simulink model "subsystem1"  (R2023a)
settings: Solver=VariableStepAuto  StartTime=0.0  StopTime=10  RelTol=1e-3  AbsTol=1e-3
values from neighbouring files (symbols this model uses):
  b = 1    [KATSAYI.m]    (also in hiz.m = 0.1; kat.m = 0.1; matlab.mat; untitled.m = 0.1)
  B1 = 1    [KATSAYI.m]    (also in hiz.m; kat.m; matlab.mat; untitled.m)
  B2 = 1    [KATSAYI.m]    (also in hiz.m; kat.m; matlab.mat; untitled.m)
  B3 = 1    [KATSAYI.m]    (also in matlab.mat; untitled.m)
  J = 1    [KATSAYI.m]    (also in hiz.m = 0.01; kat.m = 0.01; matlab.mat; untitled.m = 0.01)
  J1 = 1    [KATSAYI.m]    (also in hiz.m = 0.1; kat.m = 0.1; matlab.mat; untitled.m)
  J2 = 1    [KATSAYI.m]    (also in hiz.m = 0.1; kat.m = 0.1; matlab.mat; untitled.m)
  J3 = 1    [KATSAYI.m]    (also in matlab.mat; untitled.m)
  K = 1    [KATSAYI.m]    (also in hiz.m = 0.01; kat.m = 0.01; matlab.mat; untitled.m = 0.01)
  K1 = 1    [KATSAYI.m]    (also in hiz.m = 100; kat.m = 100; matlab.mat; untitled.m)
  K2 = 1    [KATSAYI.m]    (also in matlab.mat; untitled.m)
  K3 = 1    [KATSAYI.m]    (also in matlab.mat; untitled.m)
  L = 1    [KATSAYI.m]    (also in hiz.m = 0.5; kat.m = 0.5; matlab.mat; untitled.m = 0.5)
  R = 1    [KATSAYI.m]    (also in hiz.m; kat.m; matlab.mat; untitled.m)
  St = 2    [matlab.mat]    (also in untitled.m = 1)
libraries: fl_lib x26, nesl_utility x21, ee_lib x4, sdl_lib x3, simulink x2
(part 2 of 2)

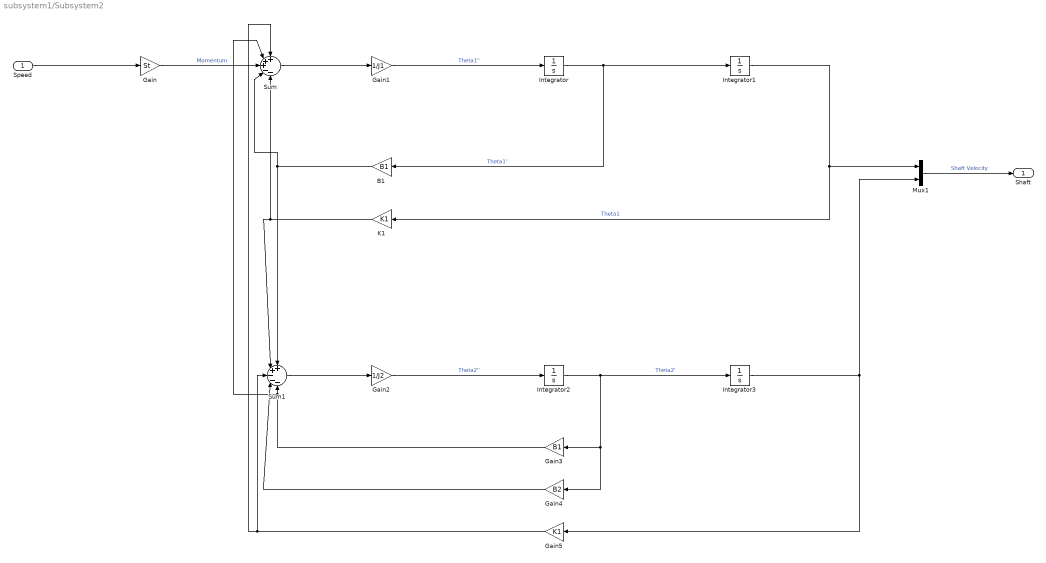
== system subsystem1/Subsystem2 ==
  Speed : Inport
  B1 : Gain  Gain=B1
  Gain : Gain  Gain=St
  Gain1 : Gain  Gain=1/J1
  Gain2 : Gain  Gain=1/J2
  Gain3 : Gain  Gain=B1
  Gain4 : Gain  Gain=B2
  Gain5 : Gain  Gain=K1
  Integrator{,1..3} (4 alike) : Integrator
  K1 : Gain  Gain=K1
  Mux1 : Mux  Inputs=2
  Sum : Sum  Inputs=+++--
  Sum1 : Sum  Inputs=++---
  Shaft : Outport
  wires:
  Mux1/1 -> Shaft/1  "Shaft Velocity"
  Speed/1 -> Gain/1
  Sum/1 -> Gain1/1
  Gain/1 -> Sum/3  "Momentum"
  Gain1/1 -> Integrator/1  "Theta1''"
  Integrator/1 -> B1/1, Integrator1/1  "Theta1'"
  B1/1 -> Sum1/1, Sum/4
  Integrator1/1 -> K1/1, Mux1/1  "Theta1"
  K1/1 -> Sum1/2, Sum/5
  Sum1/1 -> Gain2/1
  Gain2/1 -> Integrator2/1  "Theta2''"
  Integrator2/1 -> Gain4/1, Gain3/1, Integrator3/1  "Theta2'"
  Gain3/1 -> Sum/2, Sum1/5
  Gain4/1 -> Sum1/4
  Integrator3/1 -> Mux1/2, Gain5/1
  Gain5/1 -> Sum/1, Sum1/3

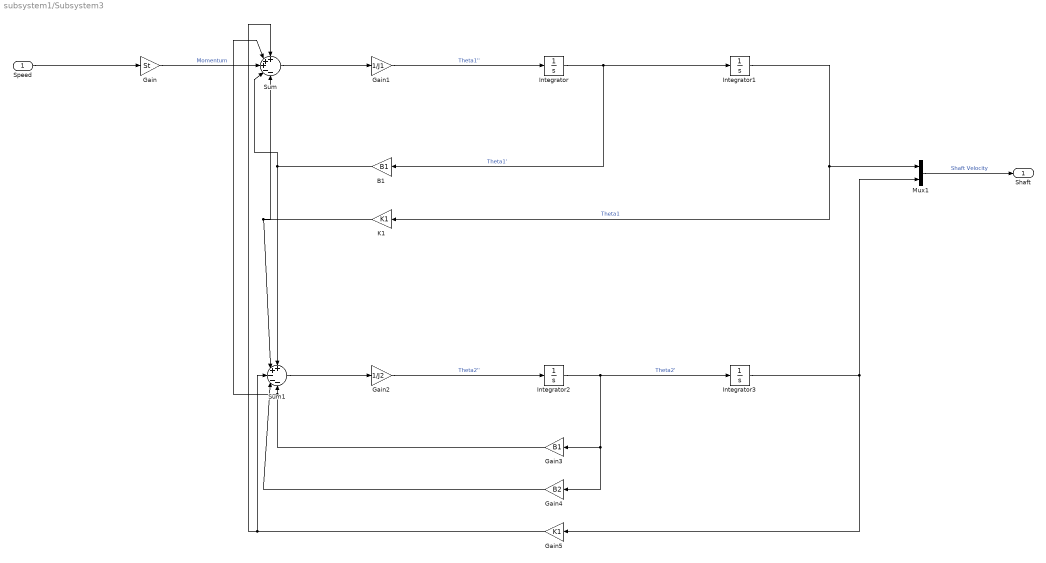
== system subsystem1/Subsystem3 ==
  Speed : Inport
  B1 : Gain  Gain=B1
  Gain : Gain  Gain=St
  Gain1 : Gain  Gain=1/J1
  Gain2 : Gain  Gain=1/J2
  Gain3 : Gain  Gain=B1
  Gain4 : Gain  Gain=B2
  Gain5 : Gain  Gain=K1
  Integrator{,1..3} (4 alike) : Integrator
  K1 : Gain  Gain=K1
  Mux1 : Mux  Inputs=2
  Sum : Sum  Inputs=+++--
  Sum1 : Sum  Inputs=++---
  Shaft : Outport
  wires:
  Gain5/1 -> Sum1/3, Sum/1
  Integrator3/1 -> Gain5/1, Mux1/2
  Gain4/1 -> Sum1/4
  Gain3/1 -> Sum1/5, Sum/2
  Integrator2/1 -> Integrator3/1, Gain3/1, Gain4/1  "Theta2'"
  Gain2/1 -> Integrator2/1  "Theta2''"
  Sum1/1 -> Gain2/1
  K1/1 -> Sum/5, Sum1/2
  Integrator1/1 -> Mux1/1, K1/1  "Theta1"
  B1/1 -> Sum/4, Sum1/1
  Integrator/1 -> Integrator1/1, B1/1  "Theta1'"
  Gain1/1 -> Integrator/1  "Theta1''"
  Gain/1 -> Sum/3  "Momentum"
  Sum/1 -> Gain1/1
  Speed/1 -> Gain/1
  Mux1/1 -> Shaft/1  "Shaft Velocity"

== system subsystem1/DC Motor Model/DC MOTOR ==
  Rotational electromechanical converter : fl_lib/Electrical/Electrical Elements/Rotational Electromechanical Converter  K=1 V*s/rad  i_specify=off  i_priority=None  i=0 A  i_nominal_specify=off  i_nominal_unit=A  i_nominal_value=1  v_specify=off  v_priority=None  v=0 V  v_nominal_specify=off  v_nominal_unit=V  v_nominal_value=1  t_specify=off  t_priority=None  t=0 N*m  t_nominal_specify=off  t_nominal_unit=N*m  t_nominal_value=1  w_specify=off  w_priority=None  w=0 rad/s  w_nominal_specify=off  w_nominal_unit=rad/s  w_nominal_value=1
  Rotational damper : fl_lib/Mechanical/Rotational Elements/Rotational Damper  D=1 N*m*s/rad  w_specify=off  w_priority=None  w=0 rad/s  w_nominal_specify=off  w_nominal_unit=rad/s  w_nominal_value=1  t_specify=off  t_priority=None  t=0 N*m  t_nominal_specify=off  t_nominal_unit=N*m  t_nominal_value=1
  inductor : ee_lib/Passive/Inductor  l=1 H  enable_L_tol=ee.enum.toleranceApplication.none  L_tol=20  tol_distribution=ee.enum.toleranceDistribution.uniform  nSigma=4  r=0 Ohm  g=1e-9 1/Ohm  enable_operating_limits=ee.enum.enable.no  operating_limit_action=ee.enum.passive.reportOpLim.warn  max_working_current=1 A  power_rating=1 W  enable_faults=ee.enum.enable.no  fault_action=simscape.enum.assert.action.none  lambdaPercent=50  k_faulted=0.9999  turnsShort=ee.enum.passive.inductor.turnsShortOption.no  openCct=ee.enum.enable.no  groundShort=ee.enum.passive.inductor.groundShortOption.no  groundShortG=0 1/Ohm  tau_fault=1e-3 s  fault_trigger=ee.enum.faults.faultTrigger.temporal  t_fault=1 s  max_permissible_voltage=100 V  n_fail_on_voltage=1  max_permissible_current=1 A  t_fail_on_current=1 s  i_L_specify=off  i_L_priority=High  i_L=0 A  i_L_nominal_specify=off  i_L_nominal_unit=A  i_L_nominal_value=1
  inertia : fl_lib/Mechanical/Rotational Elements/Inertia  inertia=0.01 kg*m^2  num_ports=foundation.enum.numPorts2.one  w_specify=off  w_priority=High  w=0 rad/s  w_nominal_specify=off  w_nominal_unit=rad/s  w_nominal_value=1  t_specify=off  t_priority=None  t=0 N*m  t_nominal_specify=off  t_nominal_unit=N*m  t_nominal_value=1
  resistor : fl_lib/Electrical/Electrical Elements/Resistor  R=1 Ohm  i_specify=off  i_priority=None  i=0 A  i_nominal_specify=off  i_nominal_unit=A  i_nominal_value=1  v_specify=off  v_priority=None  v=0 V  v_nominal_specify=off  v_nominal_unit=V  v_nominal_value=1
  V+ : PMIOPort  Side=Left
  V- : PMIOPort  Port=2  Side=Left
  R : PMIOPort  Port=3  Side=Left
  C : PMIOPort  Port=4  Side=Left
  connections:
  V+/RConn1 -- resistor/LConn1
  inductor/LConn1 -- resistor/RConn1
  Rotational electromechanical converter/RConn2 -- C/RConn1 -- Rotational damper/LConn1
  V-/RConn1 -- Rotational electromechanical converter/RConn1
  inductor/RConn1 -- Rotational electromechanical converter/LConn1
  Rotational electromechanical converter/LConn2 -- inertia/LConn1 -- Rotational damper/RConn1 -- R/RConn1

== system subsystem1/Motor Model2/Speed Load2 ==
  MRRef : fl_lib/Mechanical/Rotational Elements/Mechanical Rotational Reference
  Motion Sensor : fl_lib/Mechanical/Mechanical Sensors/Ideal Rotational Motion Sensor  reference=foundation.enum.MeasurementReference.difference  acceleration_port=true  velocity_port=true  position_port=true  wrap_angle=true  offset=0 rad
      settings: InternalSimscapePortConfiguration="{\"Bottom\":[],\"Left\":[{\"id\":\"R\",\"label\":\"R\",\"type\":\"foundation.mechanical.rotational.rotational\"}],\"Right\":[{\"id\":\"C\",\"label\":\"C\",\"type\":\"foundation.mechanical.rotational.rotational\"},{\"id\":\"alpha\",\"label\":\"α\",\"type\":\"output\"},{\"id\":\"W\",\"label\":\"W\",\"type\":\"output\"},{\"id\":\"A\",\"label\":\"A\",\"type\":\"output\"}],\"Top\":[]}"
  PS-Simulink Converter1 : nesl_utility/PS-Simulink Converter  PhysicalDomain=network_engine_domain  SubClassName=ps_output  LeftPortType=input  RightPortType=output  PseudoPeriodic=off  Frequencies=[]  VectorFormat=1-D array  Unit=rad/s  AffineConversion=off
  R : PMIOPort  Side=Left
  w : Outport  VectorParamsAs1DForOutWhenUnconnected=off
  wires:
  PS-Simulink Converter1/1 -> w/1  "Follower"
  connections:
  R/RConn1 -- Motion Sensor/LConn1
  MRRef/LConn1 -- Motion Sensor/RConn1
  Motion Sensor/RConn3 -- PS-Simulink Converter1/LConn1
